simulink model "top_level_algo"  (R2022b)
settings: Solver=FixedStepAuto  StartTime=0.0  StopTime=inf  FixedStep=1e-3  RelTol=1e-3
values from neighbouring files (symbols this model uses):
  clk_period = 8    [Cals.m]
  gear_ratio = 10    [Cals.m]
  update_rate = 0.5    [Cals.m]
  Vdd = 3    [Cals.m]
undefined symbols (not defined in the file or in its folder): sigbuilder_block
libraries: simulink x24, stm32f4xxblockslib x12, embmathops x9, arduinolib x8, dspstat3 x4, dspswit3 x2
(part 1 of 3)
settings Model: NumberOfSteps=1000  ExtModeTrigDuration=2  Creator=eahil  LastModifiedBy=eahil
settings SolverCC: AutoInsertRateTranBlk=on
settings OptimizationCC: EnhancedBackFolding=on  PassReuseOutputArgsAs=Individual arguments  ZeroExternalMemoryAtStartup=off  ZeroInternalMemoryAtStartup=off  MaxStackSize=64  OptimizeBlockOrder=speed  DifferentSizesBufferReuse=on  OptimizationCustomize=off  EfficientTunableParamExpr=on
settings DebuggingCC: ParameterTunabilityLossMsg=error  UnconnectedInputMsg=warning  UnconnectedOutputMsg=warning  UnconnectedLineMsg=warning
settings HardwareCC: ProdBitPerPointer=32  ProdBitPerSizeT=32  ProdBitPerPtrDiffT=32  ProdLargestAtomicInteger=Long  ProdLargestAtomicFloat=Double  ProdWordSize=32  ProdLongLongMode=on  ProdHWDeviceType=ARM Compatible->ARM Cortex
settings ModelReferenceCC: EnableRefExpFcnMdlSchedulingChecks=on
settings SFSimCC: MATLABDynamicMemAlloc=off
settings RTWCC: Description=Embedded Coder  SystemTargetFile=ert.tlc  HardwareBoard=STM32F4xx Based  TLCOptions=-aInlineSetEventsForThisBaseRateFcn=TLC_FALSE -aSuppressMultiTaskScheduler=TLC_FALSE -aRateBasedStepFcn=1  TemplateMakefile=ert_default_tmf  Toolchain=GNU Tools for ARM Embedded Processors  BuildConfiguration=Faster Runs  DLArmComputeVersion=19.05
settings CodeAppCC: ForceParamTrailComments=on  IgnoreCustomStorageClasses=off  OperatorAnnotations=on  SimulinkDataObjDesc=on  SFDataObjDesc=on  InsertBlockDesc=on
settings ERTTargetCC: CodeReplacementLibrary=ARM Cortex-M  SupportContinuousTime=on  ExtModeTransport=3  ExtModeStaticAlloc=on  ExtModeStaticAllocSize=2048  ExtModeMexFile=ext_xcp  ExtModeIntrfLevel=Level2 - Open

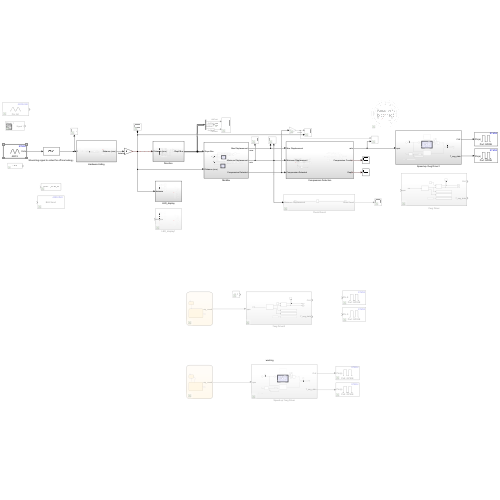
[thumbnail: Simulink's stored preview of the top-level diagram]
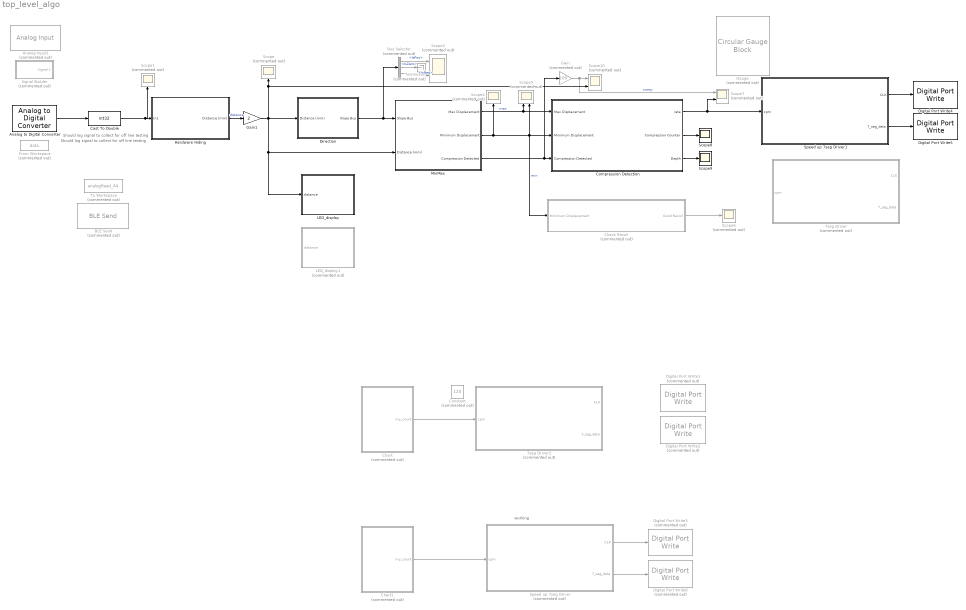
== system top_level_algo ==
  note: working
  note: Should log signal to collect for off line testing
  note: Should log signal to collect for off line testing
  7seg Driver : Subsystem  Commented=on
  7seg Driver2 : Subsystem  Commented=on
  Analog Input1 : arduinolib/Analog Input  Commented=on  pinNumber=0  ReadResultsOnly=off  ConversionTriggerSource=Software  ExternalTriggerType=uint32( 0 )  OutputDataType=uint16  EnableConversionCompleteNotify=off  EnableOuputStatus=off  SampleTime=-1  blockPlatform=arduino
  Analog to Digital Converter : stm32f4xxblockslib/Analog to Digital Converter  ADCModule=ADC3  ConversionGroup=Regular  TriggerMode=Trigger and read  NumberOfConversions=1  OutputStatus=off  SampleTime=-1  EnableSimPort=off
  BLE Send : arduinolib/BLE Send  Commented=on  DeviceMode=Peripheral (Server)  BluetoothAddress=""  CharUUID=""  ServiceUUID=""  device=No Devices  character=No Characteristics  CustomService=off  ServiceName=Generic Access  CharacteristicName=Device Name  CustomServiceUUID=<Enter Service UUID>  CustomCharUUID=<Enter Characteristic UUID>  charseruuid=<empty>  seruuid=00001810-0000-1000-8000-00805f9b34fb  chruuid=00002a00-0000-1000-8000-00805f9b34fb  PeripheralService=1800  PeripheralCharacteristic=2a00  Devicename=""  IsCustomService=0  Size=-1
  Bus Selector : BusSelector  Commented=on  OutputSignals=IsPos,IsZero,IsNeg
  Cast To Double : DataTypeConversion  OutDataTypeStr=int32  SaturateOnIntegerOverflow=off  RndMeth=Floor
  Chart : Stateflow chart  Commented=on  TreatAsAtomicUnit=on
  Chart1 : Stateflow chart  Commented=on  TreatAsAtomicUnit=on
  Check Recoil : Subsystem  Commented=on
  Compression Detection : Subsystem
  Constant : Constant  Commented=on  Value=120
  Digital Port Write1 : stm32f4xxblockslib/Digital Port Write  Commented=on  PortName=GPIOE  PinNumber=[8]  ReadOperation=off  IOAsArray=off  EnableSimPort=off
  Digital Port Write2 : stm32f4xxblockslib/Digital Port Write  Commented=on  PortName=GPIOE  PinNumber=[9]  ReadOperation=off  IOAsArray=off  EnableSimPort=off
  Digital Port Write3 : stm32f4xxblockslib/Digital Port Write  Commented=on  PortName=GPIOE  PinNumber=[8]  ReadOperation=off  IOAsArray=on  EnableSimPort=off
  Digital Port Write4 : stm32f4xxblockslib/Digital Port Write  PortName=GPIOE  PinNumber=[8]  ReadOperation=off  IOAsArray=on  EnableSimPort=off
  Digital Port Write5 : stm32f4xxblockslib/Digital Port Write  PortName=GPIOE  PinNumber=[9]  ReadOperation=off  IOAsArray=on  EnableSimPort=off
  Digital Port Write6 : stm32f4xxblockslib/Digital Port Write  Commented=on  PortName=GPIOE  PinNumber=[9]  ReadOperation=off  IOAsArray=on  EnableSimPort=off
  "Direction " : Subsystem
  From Workspace : FromWorkspace  Commented=on  VariableName=data
  Gain : Gain  Commented=on  Gain=100
  Gain1 : Gain  Gain=2
  Gauge : CircularGaugeBlock  Commented=on
  Hardware Hiding : Subsystem
  LED_display : Subsystem
  LED_display1 : Subsystem  Commented=on
  MinMax : Subsystem
  Scope{,1,4,6} (4 alike) : Scope  Commented=on
  Scope{2..3,7,10} (4 alike) : Scope  Commented=on  NumInputPorts=2
  Scope8 : Scope
  Scope9 : Scope
  Signal Builder : Subsystem  Tag=STV Subsys  Commented=on  LoadFcn=sigbuilder_block('load');  StartFcn=sigbuilder_block('start');  StopFcn=sigbuilder_block('stop');  ClipboardFcn=sigbuilder_block('clipboard');  mask(Sigbuilder block){tuvar=[0:10]}
      mask help: Simulink:masks:SigbuilderBlock_MD
      mask init:
      | if ~strcmp(get_param(bdroot(gcbh),'SimulationStatus'),'stopped') tuvar = sigbuilder_block('maskInit'); end
      settings: CopyFcn=sigbuilder_block('copy');  DeleteFcn=sigbuilder_block('delete');  ModelCloseFcn=sigbuilder_block('modelClose');  PreSaveFcn=sigbuilder_block('preSave');  PauseFcn=sigbuilder_block('pause');  ContinueFcn=sigbuilder_block('continue');  NameChangeFcn=sigbuilder_block('namechange');  OpenFcn=sigbuilder_block('open',[0 36 1152 555.6 ]);  CloseFcn=sigbuilder_block('close');
      mask Display: plot(0, 0, 100, 100,[2, 2, 32, 32, 2], [68, 8, 8, 68, 68],[32, 2], [38, 38], [32, 19, 2],[53, 60, 44], [32, 17, 17, 2],[16, 16, 31, 31]);txt = getActiveGroup(gcbh);text(2, 100, txt,'verticalAlignment', 'top');
  Speed up 7seg Driver : Subsystem  Commented=on
  Speed up 7seg Driver1 : Subsystem
  Terminator : Terminator  Commented=on
  To Workspace : ToWorkspace  Commented=on  VariableName=analogRead_A4  SaveFormat=Timeseries  SampleTime=-1
  wires:
  Hardware Hiding/1(Distance (mm)) -> Gain1/1  "distance"
  MinMax/1(Max Displacement) -> Compression Detection/1(Max Displacement), Scope3/1  "max"
  MinMax/2(Minimum Displacement) -> Check Recoil/1(Minimum Displacement), Compression Detection/2(Minimum Displacement), Scope3/2, Scope4/1  "min"
  Compression Detection/2(Compression Counter) -> Scope8/1
  "Direction "/1(Slope Bus) -> MinMax/1(Slope Bus), Bus Selector/1
  Bus Selector/1 -> Scope2/1  "<IsPos>"
  Bus Selector/3 -> Scope2/2  "<IsNeg>"
  MinMax/3(Compression Detected) -> Gain/1, Compression Detection/3(Compression Detected)
  Compression Detection/3(Depth) -> Scope9/1
  Bus Selector/2 -> Terminator/1  "<IsZero>"
  Gain/1 -> Scope7/1, Scope10/1  "comp"
  Chart/1(my_count) -> 7seg Driver2/1(cpm)
  Compression Detection/1(rate) -> Speed up 7seg Driver1/1(cpm), Scope7/2
  Cast To Double/1 -> Scope1/1, Hardware Hiding/1(In1)
  Gain1/1 -> Scope/1, Scope10/2, LED_display/1(distance), MinMax/2(Distance (mm)), "Direction "/1(Distance (mm))
  Chart1/1(my_count) -> Speed up 7seg Driver/1(cpm)
  Analog to Digital Converter/1 -> Cast To Double/1
  ? -> ?
  ? -> ?
  ? -> ?
  Check Recoil/1(Good Recoil) -> Scope6/1
  Speed up 7seg Driver1/1(CLK) -> Digital Port Write4/1
  Speed up 7seg Driver1/2(7_seg_data) -> Digital Port Write5/1
  Speed up 7seg Driver/1(CLK) -> Digital Port Write3/1
  Speed up 7seg Driver/2(7_seg_data) -> Digital Port Write6/1

== system top_level_algo/7seg Driver ==
  cpm : Inport
  Display : Display  Commented=on
      settings: Format=binary (Stored Integer)
  Display1 : Display
      settings: Format=binary (Stored Integer)
  Display2 : Display
      settings: Format=binary (Stored Integer)
  HR Encoding : Subsystem
  Pulse Generator : DiscretePulseGenerator  PulseType=Time based  Period=1  PulseWidth=0.1
  Scope12 : Scope  NumInputPorts=2
  Subsystem : Subsystem
  Value : Constant  Commented=on  Value=0x065B3F00
  CLK : Outport
  7_seg_data : Outport  Port=2
  wires:
  cpm/1 -> HR Encoding/1(data)
  Pulse Generator/1 -> Subsystem/1(Set)
  Subsystem/2(data) -> Scope12/1, 7_seg_data/1  "7_seg_data"
  HR Encoding/2(Output) -> Display2/1
  Value/1 -> Display/1
  HR Encoding/1(" ") -> Display1/1, Subsystem/2(HR)
  Subsystem/1(CLK) -> CLK/1, Scope12/2  "CLK"

== system top_level_algo/7seg Driver2 ==
  cpm : Inport
  Display : Display  Commented=on
      settings: Format=binary (Stored Integer)
  Display1 : Display
      settings: Format=binary (Stored Integer)
  Display2 : Display
      settings: Format=binary (Stored Integer)
  HR Encoding : Subsystem
  Pulse Generator : DiscretePulseGenerator  PulseType=Time based  Period=1  PulseWidth=0.1
  Scope12 : Scope  NumInputPorts=2
  Subsystem : Subsystem
  Value : Constant  Commented=on  Value=0x065B3F00
  CLK : Outport
  7_seg_data : Outport  Port=2
  wires:
  cpm/1 -> HR Encoding/1(data)
  Pulse Generator/1 -> Subsystem/1(Set)
  Subsystem/2(data) -> Scope12/1, 7_seg_data/1  "7_seg_data"
  HR Encoding/2(Output) -> Display2/1
  Value/1 -> Display/1
  HR Encoding/1(" ") -> Display1/1, Subsystem/2(HR)
  Subsystem/1(CLK) -> CLK/1, Scope12/2  "CLK"

== system top_level_algo/Check Recoil ==
  Minimum Displacement : Inport
  Compare To Constant : simulink/Logic and Bit Operations/Compare To Constant  relop=<=  const=5  OutDataTypeStr=boolean
  Good Recoil : Outport
  wires:
  Minimum Displacement/1 -> Compare To Constant/1
  Compare To Constant/1 -> Good Recoil/1

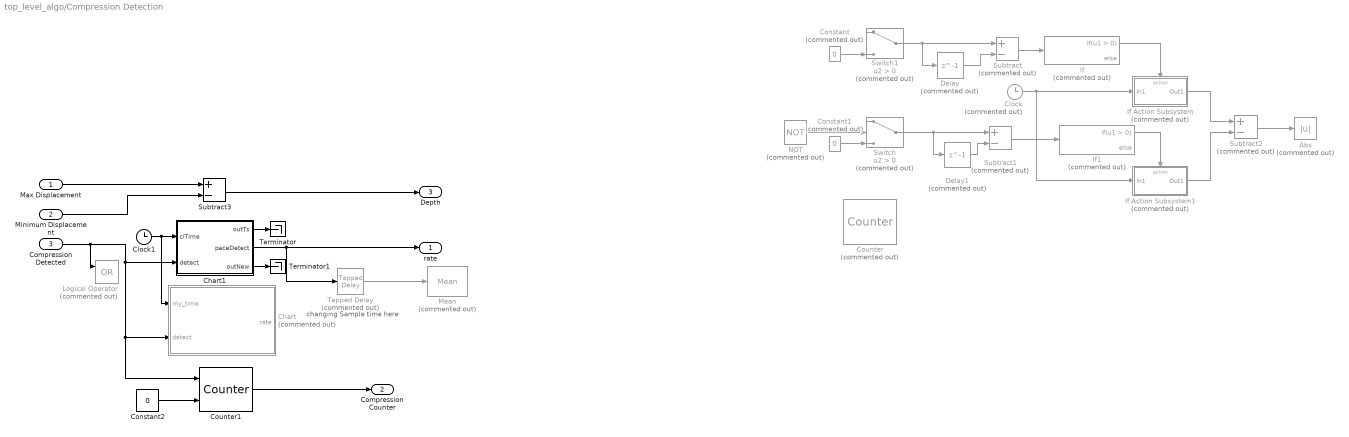
== system top_level_algo/Compression Detection ==
  note: changing Sample time here
  Max Displacement : Inport
  Minimum Displacement : Inport  Port=2
  Compression Detected : Inport  Port=3
  Abs : Abs  Commented=on  SaturateOnIntegerOverflow=off
  Chart : Stateflow chart  Commented=on  TreatAsAtomicUnit=on
  Chart1 : Stateflow chart  TreatAsAtomicUnit=on
      settings: PortSchema="{\"entries\":[{\"content\":{\"sides\":[{\"content\":{\"connectorIds\":[\"In1\",\"In2\"]},\"type\":\"ConnectorPlacement.EquallySpacedRectSide\",\"uuid\":\"de3a9b50-7e12-4e71-b702-6c1235bf285b\"},{\"content\":{\"connectorIds\":[\"Out2\",\"Out1\",\"Out3\"],\"side\":\"RIGHT\"},\"type\":\"ConnectorPlacement.EquallySpacedRectSide\",\"uuid\":\"e642841f-5679-4a41-b533-b1ac7ef5353b\"},{\"content\":{\"connectorIds\":[],\"side\":\"TOP\"},\"type\":\"ConnectorPlacement.EquallySpacedRectSide\",\"uuid\":\"59a40e31-62de-46ce-8d59-57286d1a64ca\"}]},\"type\":\"ConnectorPlacement.EquallySpacedConnector\",\"uuid\":\"d715b75a-5de9-4609-b321-1f23d868464a\"}],\"packageUris\":[\"http://schema.mathworks.com/mf0/Connector/R2020b\"],\"version\":\"1.0\"}"
  Clock : Clock  Commented=on
  Clock1 : Clock
  Constant : Constant  Commented=on  Value=0
  Constant1 : Constant  Commented=on  Value=0
  Constant2 : Constant  Value=0
  Counter : dspswit3/Counter  Commented=on  Direction=Up  CountEvent=Rising edge  CounterSize=User defined  MaxCount=255  InitialCount=0  Output=Count and Hit  HitValue=32  ResetInput=on  SamplesPerFrame=1  Ts=1  CntDtype=double  HitDtype=Logical
  Counter1 : dspswit3/Counter  Direction=Up  CountEvent=Rising edge  CounterSize=User defined  MaxCount=100  InitialCount=0  Output=Count  HitValue=32  ResetInput=on  SamplesPerFrame=1  Ts=1  CntDtype=uint16  HitDtype=Logical
  Delay : Delay  Commented=on  DelayLength=1
  Delay1 : Delay  Commented=on  DelayLength=1
  If : If  Commented=on
  If Action Subsystem : Subsystem  Commented=on  TreatAsAtomicUnit=on
  If Action Subsystem1 : Subsystem  Commented=on  TreatAsAtomicUnit=on
  If1 : If  Commented=on
  Logical Operator : Logic  Commented=on  Operator=OR  AllPortsSameDT=off  OutDataTypeStr=boolean
  Mean : dspstat3/Mean  Commented=on  run=off  InputProcessing=Columns as channels (frame based)  reset_popup=None  directionMode=Each column  dimension=1  roiEnable=off  roiType=Rectangles  roiPortion=Entire ROI  roiOutput=Individual statistics for each ROI  roiFlag=off  roundingMode=Floor  overflowMode=off  outputDataTypeStr=Inherit: Same as accumulator  outputMin=[]  outputMax=[]  outputLastDataTypeStr=Inherit: Same as accumulator
  NOT : Logic  Commented=on  Operator=NOT  IconShape=distinctive  AllPortsSameDT=off  OutDataTypeStr=boolean
  Subtract : Sum  Commented=on  Inputs=+-
  Subtract1 : Sum  Commented=on  Inputs=+-
  Subtract2 : Sum  Commented=on  Inputs=+-
  Subtract3 : Sum  Inputs=+-
  Switch : Switch  Commented=on  Criteria=u2 > Threshold  SaturateOnIntegerOverflow=off  InputSameDT=off
  Switch1 : Switch  Commented=on  Criteria=u2 > Threshold  SaturateOnIntegerOverflow=off  InputSameDT=off
  Tapped Delay : simulink/Discrete/Tapped Delay  Commented=on  vinit=0.0  samptime=0.1  NumDelays=5  DelayOrder=Oldest  includeCurrent=off
  Terminator : Terminator
  Terminator1 : Terminator
  rate : Outport
  Compression Counter : Outport  Port=2
  Depth : Outport  Port=3
  wires:
  Minimum Displacement/1 -> Subtract3/2
  Subtract1/1 -> If1/1
  Switch/1 -> Delay1/1, Subtract1/1
  Delay1/1 -> Subtract1/2
  Subtract/1 -> If/1
  Subtract2/1 -> Abs/1
  Clock/1 -> If Action Subsystem1/1(In1), If Action Subsystem/1(In1)
  If Action Subsystem/1(Out1) -> Subtract2/1
  If Action Subsystem1/1(Out1) -> Subtract2/2
  Constant/1 -> Switch1/3
  Delay/1 -> Subtract/2
  Constant1/1 -> Switch/3
  Switch1/1 -> Delay/1, Subtract/1
  If1/1 -> If Action Subsystem1/Action
  If/1 -> If Action Subsystem/Action
  NOT/1 -> Switch/2
  Max Displacement/1 -> Subtract3/1
  Subtract3/1 -> Depth/1
  Compression Detected/1 -> Logical Operator/1, Chart1/2(detect), Counter1/1, Chart/2(detect)
  Counter1/1 -> Compression Counter/1
  Constant2/1 -> Counter1/2
  Clock1/1 -> Chart/1(my_time), Chart1/1(clTime)
  Tapped Delay/1 -> Mean/1
  Chart1/1(paceDetect) -> Tapped Delay/1, rate/1
  Chart1/2(outTs) -> Terminator/1
  Chart1/3(outNew) -> Terminator1/1
  ? -> Logical Operator/2

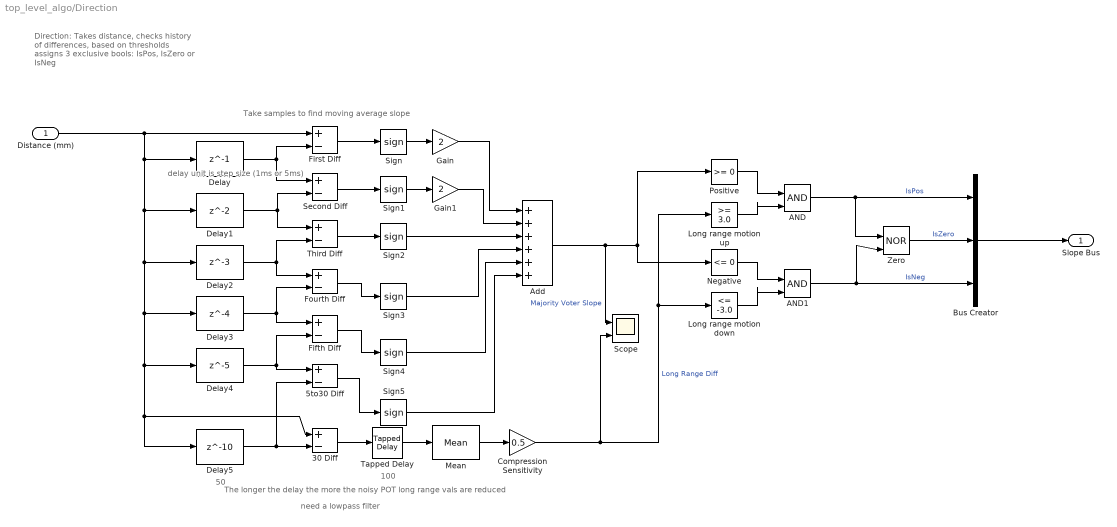
== system top_level_algo/Direction  ==
  note: 50
  note: 100
  note: need a lowpass filter
  note: The longer the delay the more the noisy POT long range vals are reduced
  note: Direction: Takes distance, checks history of differences, based on thresholds assigns 3 exclusive bools: IsPos, IsZero or IsNeg
  note: Take samples to find moving average slope
  note: delay unit is step size (1ms or 5ms)
  Distance (mm) : Inport
  30 Diff : Sum  Inputs=+-
  5to30 Diff : Sum  Inputs=+-
  AND : Logic  IconShape=distinctive  AllPortsSameDT=off  OutDataTypeStr=boolean
  AND1 : Logic  IconShape=distinctive  AllPortsSameDT=off  OutDataTypeStr=boolean
  Add : Sum  Inputs=++++++
  Bus Creator : BusCreator  Inputs=3
  Compression Sensitivity : Gain  Gain=0.5
  Delay : Delay  DelayLength=1  InputProcessing=Columns as channels (frame based)
  Delay1 : Delay  InputProcessing=Columns as channels (frame based)
  Delay2 : Delay  DelayLength=3  InputProcessing=Columns as channels (frame based)
  Delay3 : Delay  DelayLength=4  InputProcessing=Columns as channels (frame based)
  Delay4 : Delay  DelayLength=5  InputProcessing=Columns as channels (frame based)
  Delay5 : Delay  DelayLength=10  InputProcessing=Columns as channels (frame based)
  Fifth Diff : Sum  Inputs=+-
  First Diff : Sum  Inputs=+-
  Fourth Diff : Sum  Inputs=+-
  Gain : Gain  Gain=2
  Gain1 : Gain  Gain=2
  Long range motion down : simulink/Logic and Bit Operations/Compare To Constant  relop=<=  const=-3.0  OutDataTypeStr=boolean
  Long range motion up : simulink/Logic and Bit Operations/Compare To Constant  relop=>=  const=3.0  OutDataTypeStr=boolean
  Mean : dspstat3/Mean  run=off  InputProcessing=Columns as channels (frame based)  reset_popup=None  directionMode=Entire input  dimension=1  roiEnable=off  roiType=Rectangles  roiPortion=Entire ROI  roiOutput=Individual statistics for each ROI  roiFlag=off  roundingMode=Floor  overflowMode=off  outputDataTypeStr=Inherit: Same as accumulator  outputMin=[]  outputMax=[]  outputLastDataTypeStr=Inherit: Same as accumulator
  Negative : simulink/Logic and Bit Operations/Compare To Constant  relop=<=  const=0  OutDataTypeStr=boolean
  Positive : simulink/Logic and Bit Operations/Compare To Constant  relop=>=  const=0  OutDataTypeStr=boolean
  Scope : Scope  NumInputPorts=2
  Second Diff : Sum  Inputs=+-
  Sign{,1..5} (6 alike) : Signum
  Tapped Delay : simulink/Discrete/Tapped Delay  vinit=0.0  samptime=-1  NumDelays=10  DelayOrder=Oldest  includeCurrent=off
  Third Diff : Sum  Inputs=+-
  Zero : Logic  Operator=NOR  IconShape=distinctive  AllPortsSameDT=off  OutDataTypeStr=boolean
  Slope Bus : Outport
  wires:
  Sign1/1 -> Gain1/1
  Sign/1 -> Gain/1
  Second Diff/1 -> Sign1/1
  Delay1/1 -> Third Diff/1, Second Diff/2
  Third Diff/1 -> Sign2/1
  First Diff/1 -> Sign/1
  Delay/1 -> Second Diff/1, First Diff/2
  Delay2/1 -> Third Diff/2, Fourth Diff/1
  Sign2/1 -> Add/3
  Sign3/1 -> Add/4
  Fourth Diff/1 -> Sign3/1
  Delay3/1 -> Fifth Diff/1, Fourth Diff/2
  Gain/1 -> Add/1
  Gain1/1 -> Add/2
  Sign5/1 -> Add/6
  Distance (mm)/1 -> Delay5/1, 30 Diff/1, Delay4/1, Delay3/1, Delay2/1, Delay1/1, Delay/1, First Diff/1
  Delay4/1 -> 5to30 Diff/1, Fifth Diff/2
  Delay5/1 -> 5to30 Diff/2, 30 Diff/2
  5to30 Diff/1 -> Sign5/1
  Sign4/1 -> Add/5
  Fifth Diff/1 -> Sign4/1
  Add/1 -> Scope/1, Positive/1, Negative/1  "Majority Voter Slope"
  Zero/1 -> Bus Creator/2  "IsZero"
  Bus Creator/1 -> Slope Bus/1
  Positive/1 -> AND/1
  AND/1 -> Bus Creator/1, Zero/1  "IsPos"
  Long range motion up/1 -> AND/2
  AND1/1 -> Bus Creator/3, Zero/2  "IsNeg"
  Negative/1 -> AND1/1
  Long range motion down/1 -> AND1/2
  Tapped Delay/1 -> Mean/1
  Compression Sensitivity/1 -> Scope/2, Long range motion down/1, Long range motion up/1  "Long Range Diff"
  30 Diff/1 -> Tapped Delay/1
  Mean/1 -> Compression Sensitivity/1

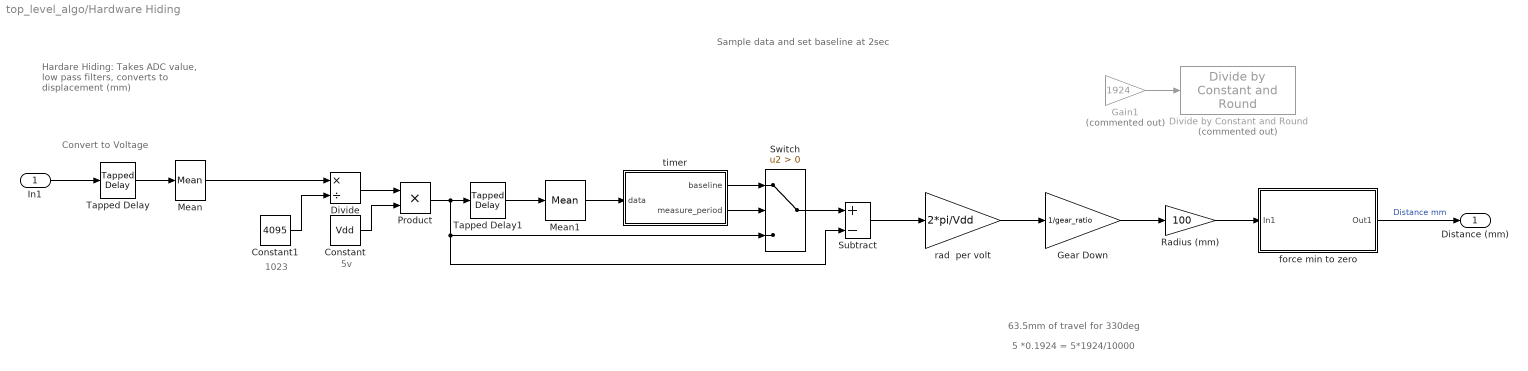
== system top_level_algo/Hardware Hiding ==
  note: 5 *0.1924 = 5*1924/10000
  note: 63.5mm of travel for 330deg
  note: 1023
  note: 5v
  note: Hardare Hiding: Takes ADC value, low pass filters, converts to displacement (mm)
  note: Sample data and set baseline at 2sec
  note: Convert to Voltage
  In1 : Inport
  Constant : Constant  Value=Vdd
  Constant1 : Constant  Value=4095  LockScale=on
  Divide : Product  Inputs=*/
  Divide by Constant and Round : embmathops/Divide by Constant and Round  Commented=on  Denominator=10000  RoundingMethod=Floor  SimulateUsing=Code generation
  Gain1 : Gain  Commented=on  Gain=1924
  Gear Down : Gain  Gain=1/gear_ratio
  Mean : dspstat3/Mean  run=off  InputProcessing=Columns as channels (frame based)  reset_popup=None  directionMode=Each column  dimension=1  roiEnable=off  roiType=Rectangles  roiPortion=Entire ROI  roiOutput=Individual statistics for each ROI  roiFlag=off  roundingMode=Floor  overflowMode=off  outputDataTypeStr=Inherit: Same as accumulator  outputMin=[]  outputMax=[]  outputLastDataTypeStr=Inherit: Same as accumulator
  Mean1 : dspstat3/Mean  run=off  InputProcessing=Columns as channels (frame based)  reset_popup=None  directionMode=Each column  dimension=1  roiEnable=off  roiType=Rectangles  roiPortion=Entire ROI  roiOutput=Individual statistics for each ROI  roiFlag=off  roundingMode=Floor  overflowMode=off  outputDataTypeStr=Inherit: Same as accumulator  outputMin=[]  outputMax=[]  outputLastDataTypeStr=Inherit: Same as accumulator
  Product : Product
  Radius (mm) : Gain  Gain=100
  Subtract : Sum  Inputs=+-
  Switch : Switch  Criteria=u2 > Threshold  SaturateOnIntegerOverflow=off  InputSameDT=off
  Tapped Delay : simulink/Discrete/Tapped Delay  vinit=0.0  samptime=0.005  NumDelays=10  DelayOrder=Oldest  includeCurrent=off
  Tapped Delay1 : simulink/Discrete/Tapped Delay  vinit=0  samptime=-1  NumDelays=20  DelayOrder=Oldest  includeCurrent=off
  force min to zero : Subsystem
  rad  per volt : Gain  Gain=2*pi/Vdd
  timer : Stateflow chart  TreatAsAtomicUnit=on
  Distance (mm) : Outport
  wires:
  Product/1 -> Subtract/2, Switch/3, Tapped Delay1/1
  timer/1(baseline) -> Switch/1
  Tapped Delay1/1 -> Mean1/1
  Mean/1 -> Divide/1
  Constant1/1 -> Divide/2
  timer/2(measure_period) -> Switch/2
  Tapped Delay/1 -> Mean/1
  Constant/1 -> Product/2
  Switch/1 -> Subtract/1
  force min to zero/1(Out1) -> Distance (mm)/1  "Distance mm"
  Divide/1 -> Product/1
  Mean1/1 -> timer/1(data)
  In1/1 -> Tapped Delay/1
  Gain1/1 -> Divide by Constant and Round/1
  ? -> Gain1/1
  Gear Down/1 -> Radius (mm)/1
  rad  per volt/1 -> Gear Down/1
  Subtract/1 -> rad  per volt/1
  Radius (mm)/1 -> force min to zero/1(In1)

== system top_level_algo/LED_display ==
  distance : Inport
  Compare To Constant : simulink/Logic and Bit Operations/Compare To Constant  relop=>  const=50  OutDataTypeStr=boolean
  Compare To Constant1 : simulink/Logic and Bit Operations/Compare To Constant  relop=>  const=40  OutDataTypeStr=boolean
  Compare To Constant2 : simulink/Logic and Bit Operations/Compare To Constant  relop=>  const=30  OutDataTypeStr=boolean
  Compare To Constant3 : simulink/Logic and Bit Operations/Compare To Constant  relop=>  const=20  OutDataTypeStr=boolean
  Compare To Constant4 : simulink/Logic and Bit Operations/Compare To Constant  relop=>  const=10  OutDataTypeStr=boolean
  Digital Port Write : stm32f4xxblockslib/Digital Port Write  PortName=GPIOE  PinNumber=[6]  ReadOperation=off  IOAsArray=on  EnableSimPort=off
  Digital Port Write1 : stm32f4xxblockslib/Digital Port Write  PortName=GPIOE  PinNumber=[5]  ReadOperation=off  IOAsArray=on  EnableSimPort=off
  Digital Port Write2 : stm32f4xxblockslib/Digital Port Write  PortName=GPIOE  PinNumber=[4]  ReadOperation=off  IOAsArray=on  EnableSimPort=off
  Digital Port Write3 : stm32f4xxblockslib/Digital Port Write  PortName=GPIOE  PinNumber=[3]  ReadOperation=off  IOAsArray=on  EnableSimPort=off
  Digital Port Write4 : stm32f4xxblockslib/Digital Port Write  PortName=GPIOE  PinNumber=[2]  ReadOperation=off  IOAsArray=on  EnableSimPort=off
  If : If  Commented=on  IfExpression=u1 > 50  ElseIfExpressions=u1 > 42, u1 >36, u1 > 28, u1 > 2
  If Action Subsystem1 : Subsystem  Commented=on  TreatAsAtomicUnit=on
  If Action Subsystem2 : Subsystem  Commented=on  TreatAsAtomicUnit=on
  If Action Subsystem3 : Subsystem  Commented=on  TreatAsAtomicUnit=on
  If Action Subsystem4 : Subsystem  Commented=on  TreatAsAtomicUnit=on
  If Action Subsystem5 : Subsystem  Commented=on  TreatAsAtomicUnit=on
  If Action Subsystem6 : Subsystem  Commented=on  TreatAsAtomicUnit=on
  wires:
  Compare To Constant2/1 -> Digital Port Write2/1
  Compare To Constant3/1 -> Digital Port Write3/1
  Compare To Constant/1 -> Digital Port Write/1
  Compare To Constant1/1 -> Digital Port Write1/1
  Compare To Constant4/1 -> Digital Port Write4/1
  If/5 -> If Action Subsystem5/Action
  ? -> If/1
  If/6 -> If Action Subsystem6/Action
  If/3 -> If Action Subsystem3/Action
  If/1 -> If Action Subsystem1/Action
  If/2 -> If Action Subsystem2/Action
  If/4 -> If Action Subsystem4/Action
  distance/1 -> Compare To Constant2/1, Compare To Constant/1, Compare To Constant1/1, Compare To Constant4/1, Compare To Constant3/1

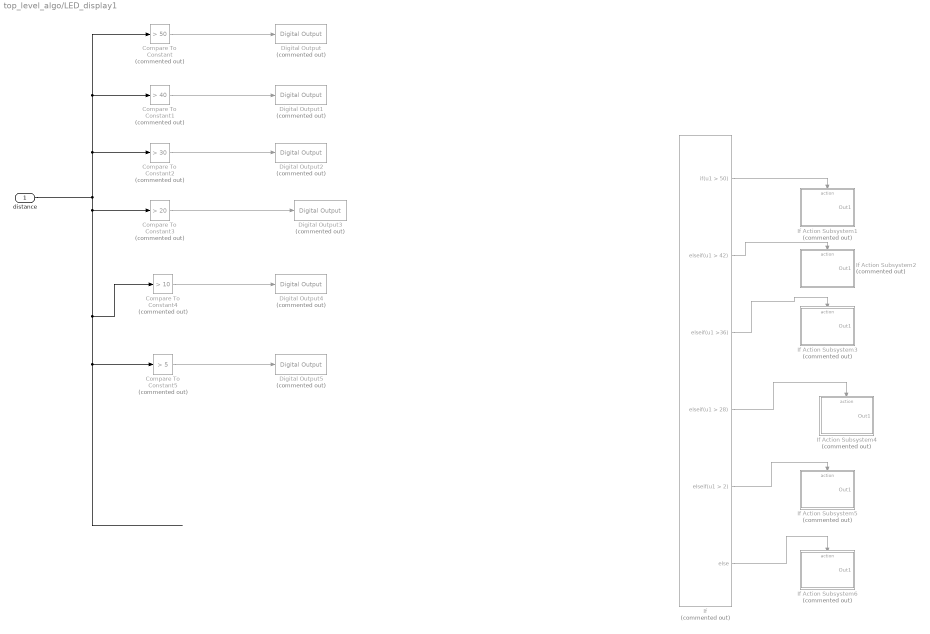
== system top_level_algo/LED_display1 ==
  distance : Inport
  Compare To Constant : simulink/Logic and Bit Operations/Compare To Constant  Commented=on  relop=>  const=50  OutDataTypeStr=boolean
  Compare To Constant1 : simulink/Logic and Bit Operations/Compare To Constant  Commented=on  relop=>  const=40  OutDataTypeStr=boolean
  Compare To Constant2 : simulink/Logic and Bit Operations/Compare To Constant  Commented=on  relop=>  const=30  OutDataTypeStr=boolean
  Compare To Constant3 : simulink/Logic and Bit Operations/Compare To Constant  Commented=on  relop=>  const=20  OutDataTypeStr=boolean
  Compare To Constant4 : simulink/Logic and Bit Operations/Compare To Constant  Commented=on  relop=>  const=10  OutDataTypeStr=boolean
  Compare To Constant5 : simulink/Logic and Bit Operations/Compare To Constant  Commented=on  relop=>  const=5  OutDataTypeStr=boolean
  Digital Output : arduinolib/Digital Output  Commented=on  pinNumber=6  Direction=output  blockPlatform=arduino
  Digital Output1 : arduinolib/Digital Output  Commented=on  pinNumber=7  Direction=output  blockPlatform=arduino
  Digital Output2 : arduinolib/Digital Output  Commented=on  pinNumber=8  Direction=output  blockPlatform=arduino
  Digital Output3 : arduinolib/Digital Output  Commented=on  pinNumber=9  Direction=output  blockPlatform=arduino
  Digital Output4 : arduinolib/Digital Output  Commented=on  pinNumber=10  Direction=output  blockPlatform=arduino
  Digital Output5 : arduinolib/Digital Output  Commented=on  pinNumber=11  Direction=output  blockPlatform=arduino
  If : If  Commented=on  IfExpression=u1 > 50  ElseIfExpressions=u1 > 42, u1 >36, u1 > 28, u1 > 2
  If Action Subsystem1 : Subsystem  Commented=on  TreatAsAtomicUnit=on
  If Action Subsystem2 : Subsystem  Commented=on  TreatAsAtomicUnit=on
  If Action Subsystem3 : Subsystem  Commented=on  TreatAsAtomicUnit=on
  If Action Subsystem4 : Subsystem  Commented=on  TreatAsAtomicUnit=on
  If Action Subsystem5 : Subsystem  Commented=on  TreatAsAtomicUnit=on
  If Action Subsystem6 : Subsystem  Commented=on  TreatAsAtomicUnit=on
  wires:
  Compare To Constant2/1 -> Digital Output2/1
  Compare To Constant3/1 -> Digital Output3/1
  Compare To Constant/1 -> Digital Output/1
  Compare To Constant1/1 -> Digital Output1/1
  Compare To Constant5/1 -> Digital Output5/1
  Compare To Constant4/1 -> Digital Output4/1
  If/5 -> If Action Subsystem5/Action
  ? -> If/1
  If/6 -> If Action Subsystem6/Action
  If/3 -> If Action Subsystem3/Action
  If/1 -> If Action Subsystem1/Action
  If/2 -> If Action Subsystem2/Action
  If/4 -> If Action Subsystem4/Action
  distance/1 -> Compare To Constant2/1, Compare To Constant/1, Compare To Constant1/1, Compare To Constant5/1, Compare To Constant4/1, Compare To Constant3/1
  ? -> ?

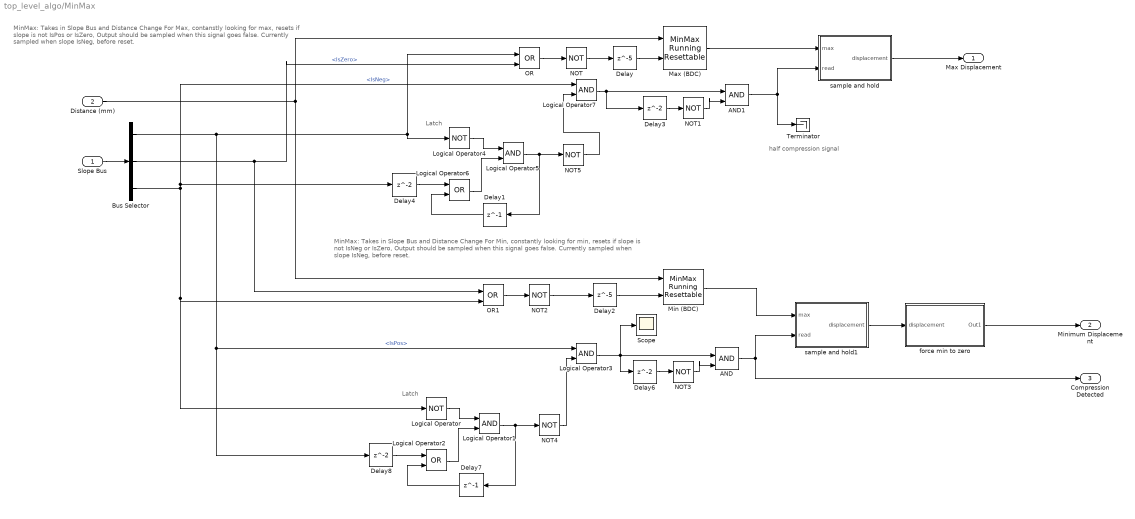
== system top_level_algo/MinMax ==
  note: half compression signal
  note: MinMax: Takes in Slope Bus and Distance Change
      | For Max, contanstly looking for max, resets if slope is not IsPos or IsZero, Output should be sampled when this signal goes false. Currently sampled when slope IsNeg, before reset.
  note: Latch
  note: MinMax: Takes in Slope Bus and Distance Change
      | For Min, constantly looking for min, resets if slope is not IsNeg or IsZero, Output should be sampled when this signal goes false. Currently sampled when slope IsNeg, before reset.
  note: Latch
  Slope Bus : Inport
  Distance (mm) : Inport  Port=2
  AND : Logic  IconShape=distinctive  AllPortsSameDT=off  OutDataTypeStr=boolean
  AND1 : Logic  IconShape=distinctive  AllPortsSameDT=off  OutDataTypeStr=boolean
  Bus Selector : BusSelector  OutputSignals=IsPos,IsZero,IsNeg
  Delay : Delay  DelayLength=5
  Delay1 : Delay  DelayLength=1
  Delay2 : Delay  DelayLength=5
  Delay3 : Delay  InitialCondition=1
  Delay4 : Delay
  Delay6 : Delay  InitialCondition=1
  Delay7 : Delay  DelayLength=1
  Delay8 : Delay
  Logical Operator : Logic  Operator=NOT  AllPortsSameDT=off  OutDataTypeStr=boolean
  Logical Operator{1,3,5,7} (4 alike) : Logic  AllPortsSameDT=off  OutDataTypeStr=boolean
  Logical Operator2 : Logic  Operator=OR  AllPortsSameDT=off  OutDataTypeStr=boolean
  Logical Operator4 : Logic  Operator=NOT  AllPortsSameDT=off  OutDataTypeStr=boolean
  Logical Operator6 : Logic  Operator=OR  AllPortsSameDT=off  OutDataTypeStr=boolean
  Max (BDC) : simulink/Math Operations/MinMax Running Resettable  Function=max  vinit=0.0
  Min (BDC) : simulink/Math Operations/MinMax Running Resettable  Function=min  vinit=100
  NOT{,1..5} (6 alike) : Logic  Operator=NOT  IconShape=distinctive  AllPortsSameDT=off  OutDataTypeStr=boolean
  OR : Logic  Operator=OR  IconShape=distinctive  AllPortsSameDT=off  OutDataTypeStr=boolean
  OR1 : Logic  Operator=OR  IconShape=distinctive  AllPortsSameDT=off  OutDataTypeStr=boolean
  Scope : Scope
  Terminator : Terminator
  force min to zero : Subsystem
  sample and hold : Stateflow chart  TreatAsAtomicUnit=on
  sample and hold1 : Stateflow chart  TreatAsAtomicUnit=on
  Max Displacement : Outport
  Minimum Displacement : Outport  Port=2
  Compression Detected : Outport  Port=3
  wires:
  Slope Bus/1 -> Bus Selector/1
  Bus Selector/1 -> OR/1, Logical Operator4/1, Delay8/1, Logical Operator3/1  "<IsPos>"
  Bus Selector/2 -> OR/2, OR1/1  "<IsZero>"
  OR/1 -> NOT/1
  NOT/1 -> Delay/1
  Max (BDC)/1 -> sample and hold/1(max)
  Delay/1 -> Max (BDC)/2
  sample and hold/1(displacement) -> Max Displacement/1
  Delay2/1 -> Min (BDC)/2
  Delay6/1 -> NOT3/1
  Min (BDC)/1 -> sample and hold1/1(max)
  Distance (mm)/1 -> Max (BDC)/1, Min (BDC)/1
  NOT2/1 -> Delay2/1
  OR1/1 -> NOT2/1
  AND/1 -> sample and hold1/2(read), Compression Detected/1
  sample and hold1/1(displacement) -> force min to zero/1(displacement)
  NOT3/1 -> AND/2
  Logical Operator1/1 -> NOT4/1, Delay7/1
  Delay7/1 -> Logical Operator2/2
  Logical Operator2/1 -> Logical Operator1/2
  Logical Operator/1 -> Logical Operator1/1
  Delay8/1 -> Logical Operator2/1
  NOT4/1 -> Logical Operator3/2
  Logical Operator3/1 -> Scope/1, AND/1, Delay6/1
  force min to zero/1(Out1) -> Minimum Displacement/1
  NOT1/1 -> AND1/2
  Delay3/1 -> NOT1/1
  AND1/1 -> Terminator/1, sample and hold/2(read)
  Delay1/1 -> Logical Operator6/2
  NOT5/1 -> Logical Operator7/2
  Logical Operator6/1 -> Logical Operator5/2
  Delay4/1 -> Logical Operator6/1
  Logical Operator5/1 -> NOT5/1, Delay1/1
  Logical Operator4/1 -> Logical Operator5/1
  Bus Selector/3 -> Delay4/1, Logical Operator7/1, OR1/2, Logical Operator/1  "<IsNeg>"
  Logical Operator7/1 -> Delay3/1, AND1/1

== system top_level_algo/Signal Builder ==
  Demux : Demux  Tag=STV Demux  Outputs=1
      settings: DisplayOption=none
  FromWs : FromWorkspace  Tag=STV FromWs  VariableName=tuvar
      SigBuilderData=|
      | common.afterFinalStr = 'Extrapolate'
      | common.sampleTime = 0
      | dataSet.timeRange = [0 10]
      | dataSet.name = 'Group 1'
      | sbobj.Groups.Name = 'Group 1'
      | sbobj.Groups.Signals.Name = 'Signal 1'
      | sbobj.Groups.Signals.XData = [0 2 2 6 6 10]
      | sbobj.Groups.Signals.YData = [0 0 1 1 0 0]
  Signal 1 : Outport  Tag=STV Outport
  wires:
  Demux/1 -> Signal 1/1
  FromWs/1 -> Demux/1

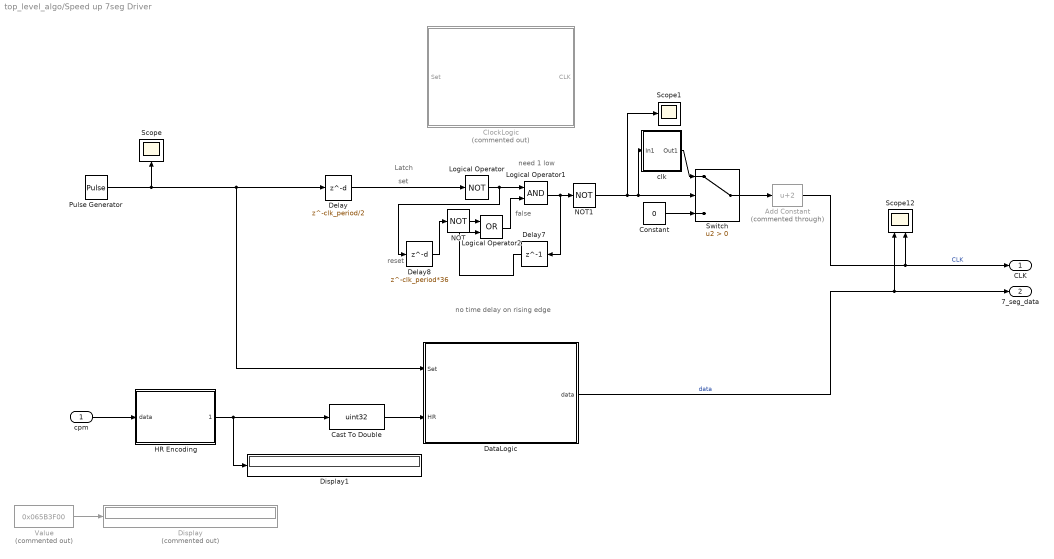
== system top_level_algo/Speed up 7seg Driver ==
  note: reset
  note: set
  note: false
  note: need 1 low
  note: Latch
  note: no time delay on rising edge
  cpm : Inport
  Add Constant : Bias  Commented=through  Bias=2  SaturateOnIntegerOverflow=off
  Cast To Double : DataTypeConversion  OutDataTypeStr=uint32  SaturateOnIntegerOverflow=off  RndMeth=Floor
  ClockLogic : Stateflow chart  Commented=on  TreatAsAtomicUnit=on
  Constant : Constant  Value=0
  DataLogic : Stateflow chart  TreatAsAtomicUnit=on
      settings: PortSchema="{\"entries\":[{\"content\":{\"sides\":[{\"content\":{\"connectorIds\":[\"In2\",\"In1\"]},\"type\":\"ConnectorPlacement.EquallySpacedRectSide\",\"uuid\":\"4f23318f-6912-4c0c-9d33-643c1a92e835\"},{\"content\":{\"connectorIds\":[\"Out1\"],\"side\":\"RIGHT\"},\"type\":\"ConnectorPlacement.EquallySpacedRectSide\",\"uuid\":\"fb7ed84c-55c8-499b-b1c5-e6b2ea6fec65\"},{\"content\":{\"connectorIds\":[],\"side\":\"TOP\"},\"type\":\"ConnectorPlacement.EquallySpacedRectSide\",\"uuid\":\"7f67bbc6-bcff-470e-a8fc-5e94445d0a2a\"}]},\"type\":\"ConnectorPlacement.EquallySpacedConnector\",\"uuid\":\"1fe3f03b-7187-41bc-b70b-9d5872e37b8d\"}],\"packageUris\":[\"http://schema.mathworks.com/mf0/Connector/R2020b\"],\"version\":\"1.0\"}"
  Delay : Delay  DelayLength=clk_period/2
  Delay7 : Delay  DelayLength=1
  Delay8 : Delay  DelayLength=clk_period*36
  Display : Display  Commented=on
      settings: Format=binary (Stored Integer)
  Display1 : Display
      settings: Format=binary (Stored Integer)
  HR Encoding : Subsystem
  Logical Operator : Logic  Operator=NOT  AllPortsSameDT=off  OutDataTypeStr=boolean
  Logical Operator1 : Logic  AllPortsSameDT=off  OutDataTypeStr=boolean
  Logical Operator2 : Logic  Operator=OR  AllPortsSameDT=off  OutDataTypeStr=boolean
  NOT : Logic  Operator=NOT  IconShape=distinctive  AllPortsSameDT=off  OutDataTypeStr=boolean
  NOT1 : Logic  Operator=NOT  IconShape=distinctive  AllPortsSameDT=off  OutDataTypeStr=boolean
  Pulse Generator : DiscretePulseGenerator  PulseType=Time based  Period=update_rate  PulseWidth=1/update_rate  PhaseDelay=2
  Scope : Scope
  Scope1 : Scope
  Scope12 : Scope  NumInputPorts=2
  Switch : Switch  Criteria=u2 > Threshold  SaturateOnIntegerOverflow=off  InputSameDT=off
  Value : Constant  Commented=on  Value=0x065B3F00
  clk : Subsystem
  CLK : Outport
  7_seg_data : Outport  Port=2
  wires:
  cpm/1 -> HR Encoding/1(data)
  Value/1 -> Display/1
  Add Constant/1 -> CLK/1, Scope12/2  "CLK"
  Logical Operator2/1 -> Logical Operator1/2
  Delay7/1 -> Logical Operator2/2
  Logical Operator1/1 -> Delay7/1, NOT1/1
  Logical Operator/1 -> Delay8/1, Logical Operator1/1
  NOT1/1 -> Scope1/1, Switch/2, clk/1(In1)
  Delay/1 -> Logical Operator/1
  Cast To Double/1 -> DataLogic/1(HR)
  Constant/1 -> Switch/3
  clk/1(Out1) -> Switch/1
  Switch/1 -> Add Constant/1
  NOT/1 -> Logical Operator2/1
  HR Encoding/1(" ") -> Display1/1, Cast To Double/1
  Pulse Generator/1 -> DataLogic/2(Set), Delay/1, Scope/1
  DataLogic/1(data) -> Scope12/1, 7_seg_data/1  "data"
  Delay8/1 -> NOT/1

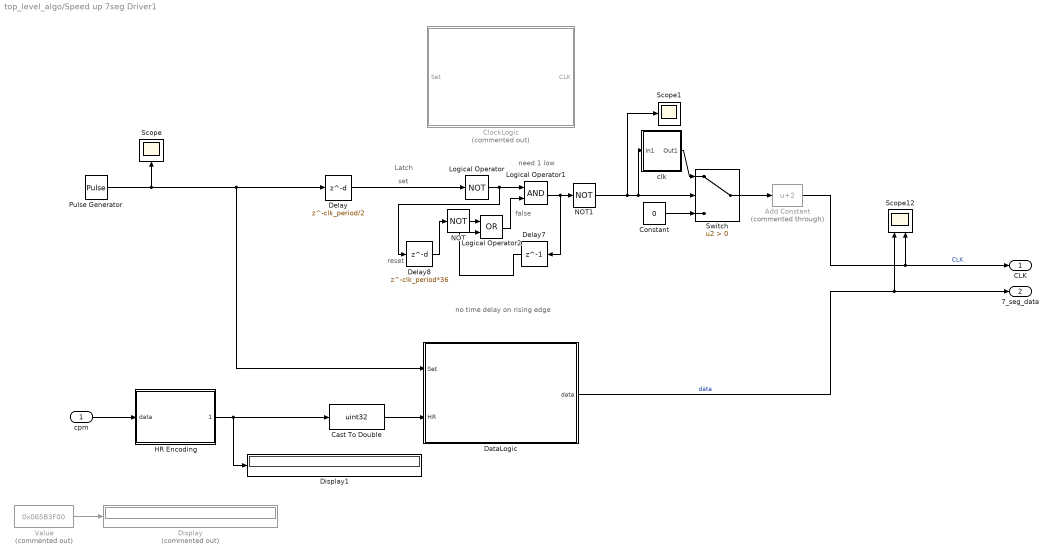
== system top_level_algo/Speed up 7seg Driver1 ==
  note: no time delay on rising edge
  note: Latch
  note: need 1 low
  note: false
  note: set
  note: reset
  cpm : Inport
  Add Constant : Bias  Commented=through  Bias=2  SaturateOnIntegerOverflow=off
  Cast To Double : DataTypeConversion  OutDataTypeStr=uint32  SaturateOnIntegerOverflow=off  RndMeth=Floor
  ClockLogic : Stateflow chart  Commented=on  TreatAsAtomicUnit=on
  Constant : Constant  Value=0
  DataLogic : Stateflow chart  TreatAsAtomicUnit=on
      settings: PortSchema="{\"entries\":[{\"content\":{\"sides\":[{\"content\":{\"connectorIds\":[\"In2\",\"In1\"]},\"type\":\"ConnectorPlacement.EquallySpacedRectSide\",\"uuid\":\"4f23318f-6912-4c0c-9d33-643c1a92e835\"},{\"content\":{\"connectorIds\":[\"Out1\"],\"side\":\"RIGHT\"},\"type\":\"ConnectorPlacement.EquallySpacedRectSide\",\"uuid\":\"fb7ed84c-55c8-499b-b1c5-e6b2ea6fec65\"},{\"content\":{\"connectorIds\":[],\"side\":\"TOP\"},\"type\":\"ConnectorPlacement.EquallySpacedRectSide\",\"uuid\":\"7f67bbc6-bcff-470e-a8fc-5e94445d0a2a\"}]},\"type\":\"ConnectorPlacement.EquallySpacedConnector\",\"uuid\":\"1fe3f03b-7187-41bc-b70b-9d5872e37b8d\"}],\"packageUris\":[\"http://schema.mathworks.com/mf0/Connector/R2020b\"],\"version\":\"1.0\"}"
  Delay : Delay  DelayLength=clk_period/2
  Delay7 : Delay  DelayLength=1
  Delay8 : Delay  DelayLength=clk_period*36
  Display : Display  Commented=on
      settings: Format=binary (Stored Integer)
  Display1 : Display
      settings: Format=binary (Stored Integer)
  HR Encoding : Subsystem
  Logical Operator : Logic  Operator=NOT  AllPortsSameDT=off  OutDataTypeStr=boolean
  Logical Operator1 : Logic  AllPortsSameDT=off  OutDataTypeStr=boolean
  Logical Operator2 : Logic  Operator=OR  AllPortsSameDT=off  OutDataTypeStr=boolean
  NOT : Logic  Operator=NOT  IconShape=distinctive  AllPortsSameDT=off  OutDataTypeStr=boolean
  NOT1 : Logic  Operator=NOT  IconShape=distinctive  AllPortsSameDT=off  OutDataTypeStr=boolean
  Pulse Generator : DiscretePulseGenerator  PulseType=Time based  Period=update_rate  PulseWidth=1/update_rate  PhaseDelay=2
  Scope : Scope
  Scope1 : Scope
  Scope12 : Scope  NumInputPorts=2
  Switch : Switch  Criteria=u2 > Threshold  SaturateOnIntegerOverflow=off  InputSameDT=off
  Value : Constant  Commented=on  Value=0x065B3F00
  clk : Subsystem
  CLK : Outport
  7_seg_data : Outport  Port=2
  wires:
  Delay8/1 -> NOT/1
  DataLogic/1(data) -> 7_seg_data/1, Scope12/1  "data"
  Pulse Generator/1 -> Scope/1, Delay/1, DataLogic/2(Set)
  HR Encoding/1(" ") -> Cast To Double/1, Display1/1
  NOT/1 -> Logical Operator2/1
  Switch/1 -> Add Constant/1
  clk/1(Out1) -> Switch/1
  Constant/1 -> Switch/3
  Cast To Double/1 -> DataLogic/1(HR)
  Delay/1 -> Logical Operator/1
  NOT1/1 -> clk/1(In1), Switch/2, Scope1/1
  Logical Operator/1 -> Logical Operator1/1, Delay8/1
  Logical Operator1/1 -> NOT1/1, Delay7/1
  Delay7/1 -> Logical Operator2/2
  Logical Operator2/1 -> Logical Operator1/2
  Add Constant/1 -> Scope12/2, CLK/1  "CLK"
  Value/1 -> Display/1
  cpm/1 -> HR Encoding/1(data)

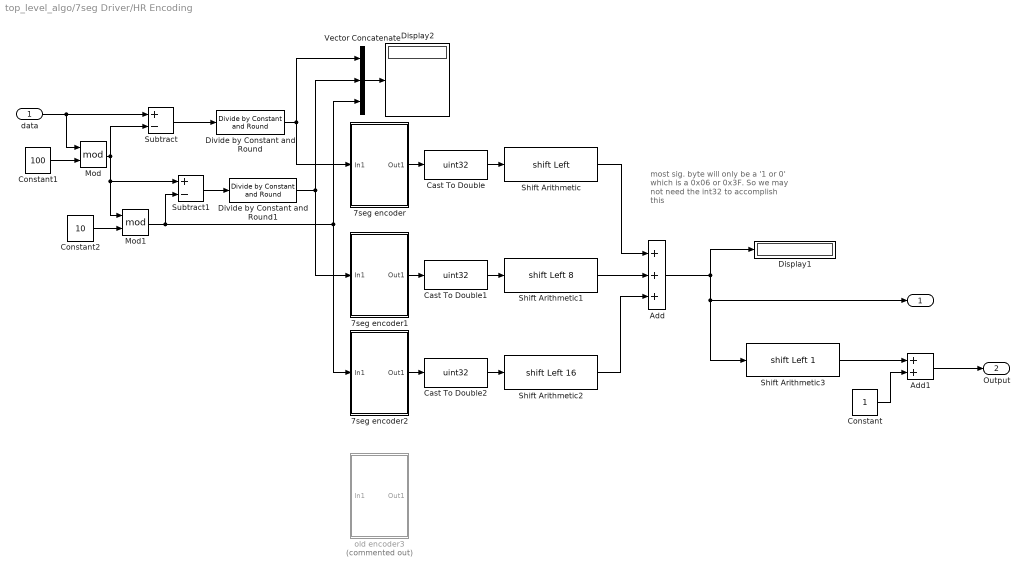
== system top_level_algo/7seg Driver/HR Encoding ==
  note: most sig. byte will only be a '1 or 0' which is a 0x06 or 0x3F. So we may not need the int32 to accomplish this
  data : Inport
  7seg encoder : Subsystem
  7seg encoder1 : Subsystem
  7seg encoder2 : Subsystem
  Add : Sum  Inputs=+++
  Add1 : Sum
  Cast To Double : DataTypeConversion  OutDataTypeStr=uint32  SaturateOnIntegerOverflow=off  RndMeth=Floor
  Cast To Double1 : DataTypeConversion  OutDataTypeStr=uint32  SaturateOnIntegerOverflow=off  RndMeth=Floor
  Cast To Double2 : DataTypeConversion  OutDataTypeStr=uint32  SaturateOnIntegerOverflow=off  RndMeth=Floor
  Constant : Constant  OutDataTypeStr=uint32
  Constant1 : Constant  Value=100
  Constant2 : Constant  Value=10
  Display1 : Display
      settings: Format=hex (Stored Integer)
  Display2 : Display
  Divide by Constant and Round : embmathops/Divide by Constant and Round  Denominator=100  RoundingMethod=Floor  SimulateUsing=Code generation
  Divide by Constant and Round1 : embmathops/Divide by Constant and Round  Denominator=10  RoundingMethod=Floor  SimulateUsing=Code generation
  Mod : Math  Operator=mod
  Mod1 : Math  Operator=mod
  Shift Arithmetic : ArithShift  BitShiftDirection=Left
  Shift Arithmetic1 : ArithShift  BitShiftNumber=8  BitShiftDirection=Left
  Shift Arithmetic2 : ArithShift  BitShiftNumber=16  BitShiftDirection=Left
  Shift Arithmetic3 : ArithShift  BitShiftNumber=1  BitShiftDirection=Left
  Subtract : Sum  Inputs=+-
  Subtract1 : Sum  Inputs=+-
  Vector Concatenate : Concatenate  NumInputs=3
  old encoder3 : Subsystem  Commented=on
  " " : Outport
  Output : Outport  Port=2
  wires:
  Shift Arithmetic1/1 -> Add/2
  Mod1/1 -> Subtract1/2, Vector Concatenate/3, 7seg encoder2/1(In1)
  Mod/1 -> Subtract/2, Subtract1/1, Mod1/1
  7seg encoder/1(Out1) -> Cast To Double/1
  Subtract/1 -> Divide by Constant and Round/1
  Constant1/1 -> Mod/2
  Divide by Constant and Round/1 -> 7seg encoder/1(In1), Vector Concatenate/1
  Subtract1/1 -> Divide by Constant and Round1/1
  Cast To Double1/1 -> Shift Arithmetic1/1
  data/1 -> Mod/1, Subtract/1
  Add/1 -> Display1/1, Shift Arithmetic3/1, " "/1
  Cast To Double/1 -> Shift Arithmetic/1
  Constant2/1 -> Mod1/2
  Vector Concatenate/1 -> Display2/1
  7seg encoder1/1(Out1) -> Cast To Double1/1
  Shift Arithmetic/1 -> Add/1
  Divide by Constant and Round1/1 -> Vector Concatenate/2, 7seg encoder1/1(In1)
  Shift Arithmetic2/1 -> Add/3
  7seg encoder2/1(Out1) -> Cast To Double2/1
  Cast To Double2/1 -> Shift Arithmetic2/1
  Constant/1 -> Add1/2
  Shift Arithmetic3/1 -> Add1/1
  Add1/1 -> Output/1

== system top_level_algo/7seg Driver/Subsystem ==
  Set : Inport
  HR : Inport  Port=2
  Add Constant : Bias  Commented=on  Bias=2  SaturateOnIntegerOverflow=off
  Cast To Double : DataTypeConversion  OutDataTypeStr=uint32  SaturateOnIntegerOverflow=off  RndMeth=Floor
  ClockLogic : Stateflow chart  TreatAsAtomicUnit=on
  DataLogic : Stateflow chart  TreatAsAtomicUnit=on
      settings: PortSchema="{\"entries\":[{\"content\":{\"sides\":[{\"content\":{\"connectorIds\":[\"In2\",\"In1\"]},\"type\":\"ConnectorPlacement.EquallySpacedRectSide\",\"uuid\":\"4f23318f-6912-4c0c-9d33-643c1a92e835\"},{\"content\":{\"connectorIds\":[\"Out1\"],\"side\":\"RIGHT\"},\"type\":\"ConnectorPlacement.EquallySpacedRectSide\",\"uuid\":\"fb7ed84c-55c8-499b-b1c5-e6b2ea6fec65\"},{\"content\":{\"connectorIds\":[],\"side\":\"TOP\"},\"type\":\"ConnectorPlacement.EquallySpacedRectSide\",\"uuid\":\"7f67bbc6-bcff-470e-a8fc-5e94445d0a2a\"}]},\"type\":\"ConnectorPlacement.EquallySpacedConnector\",\"uuid\":\"1fe3f03b-7187-41bc-b70b-9d5872e37b8d\"}],\"packageUris\":[\"http://schema.mathworks.com/mf0/Connector/R2020b\"],\"version\":\"1.0\"}"
  CLK : Outport
  data : Outport  Port=2
  wires:
  Set/1 -> DataLogic/2(Set), ClockLogic/1(Set)
  Cast To Double/1 -> DataLogic/1(HR)
  ClockLogic/1(CLK) -> CLK/1  "CLK"
  DataLogic/1(data) -> data/1  "data"
  HR/1 -> Cast To Double/1

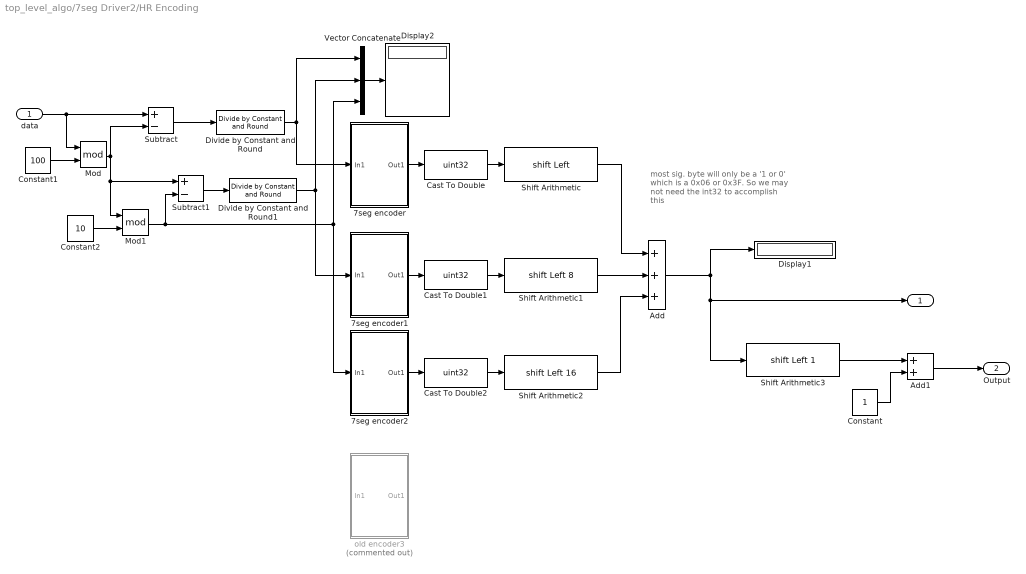
== system top_level_algo/7seg Driver2/HR Encoding ==
  note: most sig. byte will only be a '1 or 0' which is a 0x06 or 0x3F. So we may not need the int32 to accomplish this
  data : Inport
  7seg encoder : Subsystem
  7seg encoder1 : Subsystem
  7seg encoder2 : Subsystem
  Add : Sum  Inputs=+++
  Add1 : Sum
  Cast To Double : DataTypeConversion  OutDataTypeStr=uint32  SaturateOnIntegerOverflow=off  RndMeth=Floor
  Cast To Double1 : DataTypeConversion  OutDataTypeStr=uint32  SaturateOnIntegerOverflow=off  RndMeth=Floor
  Cast To Double2 : DataTypeConversion  OutDataTypeStr=uint32  SaturateOnIntegerOverflow=off  RndMeth=Floor
  Constant : Constant  OutDataTypeStr=uint32
  Constant1 : Constant  Value=100
  Constant2 : Constant  Value=10
  Display1 : Display
      settings: Format=hex (Stored Integer)
  Display2 : Display
  Divide by Constant and Round : embmathops/Divide by Constant and Round  Denominator=100  RoundingMethod=Floor  SimulateUsing=Code generation
  Divide by Constant and Round1 : embmathops/Divide by Constant and Round  Denominator=10  RoundingMethod=Floor  SimulateUsing=Code generation
  Mod : Math  Operator=mod
  Mod1 : Math  Operator=mod
  Shift Arithmetic : ArithShift  BitShiftDirection=Left
  Shift Arithmetic1 : ArithShift  BitShiftNumber=8  BitShiftDirection=Left
  Shift Arithmetic2 : ArithShift  BitShiftNumber=16  BitShiftDirection=Left
  Shift Arithmetic3 : ArithShift  BitShiftNumber=1  BitShiftDirection=Left
  Subtract : Sum  Inputs=+-
  Subtract1 : Sum  Inputs=+-
  Vector Concatenate : Concatenate  NumInputs=3
  old encoder3 : Subsystem  Commented=on
  " " : Outport
  Output : Outport  Port=2
  wires:
  Shift Arithmetic1/1 -> Add/2
  Mod1/1 -> Subtract1/2, Vector Concatenate/3, 7seg encoder2/1(In1)
  Mod/1 -> Subtract/2, Subtract1/1, Mod1/1
  7seg encoder/1(Out1) -> Cast To Double/1
  Subtract/1 -> Divide by Constant and Round/1
  Constant1/1 -> Mod/2
  Divide by Constant and Round/1 -> 7seg encoder/1(In1), Vector Concatenate/1
  Subtract1/1 -> Divide by Constant and Round1/1
  Cast To Double1/1 -> Shift Arithmetic1/1
  data/1 -> Mod/1, Subtract/1
  Add/1 -> Display1/1, Shift Arithmetic3/1, " "/1
  Cast To Double/1 -> Shift Arithmetic/1
  Constant2/1 -> Mod1/2
  Vector Concatenate/1 -> Display2/1
  7seg encoder1/1(Out1) -> Cast To Double1/1
  Shift Arithmetic/1 -> Add/1
  Divide by Constant and Round1/1 -> Vector Concatenate/2, 7seg encoder1/1(In1)
  Shift Arithmetic2/1 -> Add/3
  7seg encoder2/1(Out1) -> Cast To Double2/1
  Cast To Double2/1 -> Shift Arithmetic2/1
  Constant/1 -> Add1/2
  Shift Arithmetic3/1 -> Add1/1
  Add1/1 -> Output/1

== system top_level_algo/7seg Driver2/Subsystem ==
  Set : Inport
  HR : Inport  Port=2
  Add Constant : Bias  Bias=2  SaturateOnIntegerOverflow=off
  Cast To Double : DataTypeConversion  OutDataTypeStr=uint32  SaturateOnIntegerOverflow=off  RndMeth=Floor
  ClockLogic : Stateflow chart  TreatAsAtomicUnit=on
  DataLogic : Stateflow chart  TreatAsAtomicUnit=on
      settings: PortSchema="{\"entries\":[{\"content\":{\"sides\":[{\"content\":{\"connectorIds\":[\"In2\",\"In1\"]},\"type\":\"ConnectorPlacement.EquallySpacedRectSide\",\"uuid\":\"4f23318f-6912-4c0c-9d33-643c1a92e835\"},{\"content\":{\"connectorIds\":[\"Out1\"],\"side\":\"RIGHT\"},\"type\":\"ConnectorPlacement.EquallySpacedRectSide\",\"uuid\":\"fb7ed84c-55c8-499b-b1c5-e6b2ea6fec65\"},{\"content\":{\"connectorIds\":[],\"side\":\"TOP\"},\"type\":\"ConnectorPlacement.EquallySpacedRectSide\",\"uuid\":\"7f67bbc6-bcff-470e-a8fc-5e94445d0a2a\"}]},\"type\":\"ConnectorPlacement.EquallySpacedConnector\",\"uuid\":\"1fe3f03b-7187-41bc-b70b-9d5872e37b8d\"}],\"packageUris\":[\"http://schema.mathworks.com/mf0/Connector/R2020b\"],\"version\":\"1.0\"}"
  CLK : Outport
  data : Outport  Port=2
  wires:
  Set/1 -> DataLogic/2(Set), ClockLogic/1(Set)
  Cast To Double/1 -> DataLogic/1(HR)
  ClockLogic/1(CLK) -> Add Constant/1  "CLK"
  DataLogic/1(data) -> data/1  "data"
  HR/1 -> Cast To Double/1
  Add Constant/1 -> CLK/1

== system top_level_algo/Compression Detection/If Action Subsystem ==
  In1 : Inport
  Action Port : ActionPort  ActionPortLabel=if(u1 > 0)
  Out1 : Outport
  wires:
  In1/1 -> Out1/1

== system top_level_algo/Compression Detection/If Action Subsystem1 ==
  In1 : Inport
  Action Port : ActionPort  ActionPortLabel=if(u1 > 0)
  Out1 : Outport
  wires:
  In1/1 -> Out1/1

== system top_level_algo/Hardware Hiding/force min to zero ==
  In1 : Inport
  Constant : Constant  Value=0
  If : If  IfExpression=u1 < 0
  If Action Subsystem : Subsystem  TreatAsAtomicUnit=on
  If Action Subsystem1 : Subsystem  TreatAsAtomicUnit=on
  Merge : Merge
  Out1 : Outport
  wires:
  Merge/1 -> Out1/1
  If Action Subsystem1/1(Out1) -> Merge/2
  If Action Subsystem/1(Out1) -> Merge/1
  If/2 -> If Action Subsystem1/Action
  If/1 -> If Action Subsystem/Action
  In1/1 -> If Action Subsystem1/1(In1), If/1
  Constant/1 -> If Action Subsystem/1(In1)

== system top_level_algo/LED_display/If Action Subsystem1 ==
  Action Port : ActionPort  ActionPortLabel=if(u1 > 50)
  Constant : Constant  Value=0x3F
  Out1 : Outport
  wires:
  Constant/1 -> Out1/1

== system top_level_algo/LED_display/If Action Subsystem2 ==
  Action Port : ActionPort  ActionPortLabel=elseif(u1 > 42)
  Constant : Constant  Value=0x06
  Out1 : Outport
  wires:
  Constant/1 -> Out1/1

== system top_level_algo/LED_display/If Action Subsystem3 ==
  Action Port : ActionPort  ActionPortLabel=elseif( u1 >36)
  Constant : Constant  Value=0x5B
  Out1 : Outport
  wires:
  Constant/1 -> Out1/1

== system top_level_algo/LED_display/If Action Subsystem4 ==
  Action Port : ActionPort  ActionPortLabel=elseif( u1 > 28)
  Constant : Constant  Value=0x4F
  Out1 : Outport
  wires:
  Constant/1 -> Out1/1

== system top_level_algo/LED_display/If Action Subsystem5 ==
  Action Port : ActionPort  ActionPortLabel=elseif( u1 > 2)
  Constant : Constant  Value=0x66
  Out1 : Outport
  wires:
  Constant/1 -> Out1/1

== system top_level_algo/LED_display/If Action Subsystem6 ==
  Action Port : ActionPort  ActionPortLabel=else
  Constant : Constant  Value=0x6D
  Out1 : Outport
  wires:
  Constant/1 -> Out1/1

== system top_level_algo/LED_display1/If Action Subsystem1 ==
  Action Port : ActionPort
  Constant : Constant  Value=0x3F
  Out1 : Outport
  wires:
  Constant/1 -> Out1/1

== system top_level_algo/LED_display1/If Action Subsystem2 ==
  Action Port : ActionPort
  Constant : Constant  Value=0x06
  Out1 : Outport
  wires:
  Constant/1 -> Out1/1

== system top_level_algo/LED_display1/If Action Subsystem3 ==
  Action Port : ActionPort
  Constant : Constant  Value=0x5B
  Out1 : Outport
  wires:
  Constant/1 -> Out1/1

== system top_level_algo/LED_display1/If Action Subsystem4 ==
  Action Port : ActionPort
  Constant : Constant  Value=0x4F
  Out1 : Outport
  wires:
  Constant/1 -> Out1/1

== system top_level_algo/LED_display1/If Action Subsystem5 ==
  Action Port : ActionPort
  Constant : Constant  Value=0x66
  Out1 : Outport
  wires:
  Constant/1 -> Out1/1

== system top_level_algo/LED_display1/If Action Subsystem6 ==
  Action Port : ActionPort
  Constant : Constant  Value=0x6D
  Out1 : Outport
  wires:
  Constant/1 -> Out1/1

== system top_level_algo/MinMax/force min to zero ==
  displacement : Inport
  Constant : Constant  Value=0
  If : If  IfExpression=u1 < 0
  If Action Subsystem : Subsystem  TreatAsAtomicUnit=on
  If Action Subsystem1 : Subsystem  TreatAsAtomicUnit=on
  Merge : Merge
  Out1 : Outport
  wires:
  Merge/1 -> Out1/1
  If Action Subsystem1/1(Out1) -> Merge/2
  If Action Subsystem/1(Out1) -> Merge/1
  If/2 -> If Action Subsystem1/Action
  If/1 -> If Action Subsystem/Action
  displacement/1 -> If Action Subsystem1/1(In1), If/1
  Constant/1 -> If Action Subsystem/1(In1)
